simulink model "sfcndemo_vsfunc"  (Simulink 7.6)
settings: Solver=ode45  StartTime=0.0  StopTime=50  RelTol=1e-3
Description:
  | Continuous-Time Variable Step S-function
settings Model: Creator=The MathWorks Inc.  ExtModeTrigMode=oneshot  ExtModeArmWhenConnect=off  ExtModeAutoUpdateStatusClock=off
settings DataIOCC: LimitDataPoints=off  SaveFormat=StructureWithTime  SaveState=on  OutputSaveName=yout1
settings OptimizationCC: BlockReduction=off  BooleanDataType=off  InlineInvariantSignals=on  InitFltsAndDblsToZero=on
settings DebuggingCC: SaveWithParameterizedLinksMsg=none  SignalResolutionControl=TryResolveAllWithWarning  SolverPrmCheckMsg=none  MultiTaskDSMMsg=warning  MultiTaskCondExecSysMsg=none
settings HardwareCC: TargetUnknown=on
settings RTWCC: IncludeERTFirstTime=on
settings CodeAppCC: CustomSymbolStrFcn=$F$N$M
settings GRTTargetCC: TargetFcnLib=ansi_tfl_tmw.mat

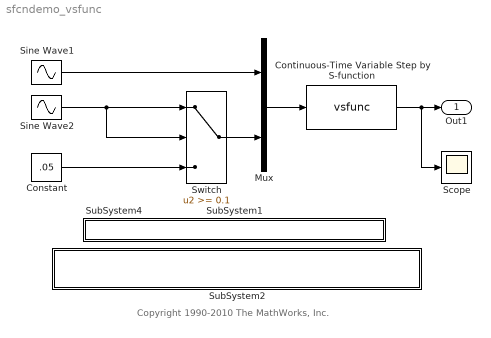
== system sfcndemo_vsfunc ==
  note: Copyright 1990-2010 The MathWorks, Inc.
  Constant : Constant  Value=.05
  Continuous-Time Variable Step by S-function : S-Function  FunctionName=vsfunc  EnableBusSupport=off
      mask Display: disp('dt           = u(2)\ny(t + dt) = u(t)')
  Mux : Mux  Inputs=2
  Scope : Scope
      settings: TimeRange=50  YMin=-1  YMax=1  SaveName=scopeout1
  Sine Wave1 : Sin  Frequency=2*pi  SampleTime=0
  Sine Wave2 : Sin  Amplitude=2  Frequency=2*pi  SampleTime=0
  SubSystem1 : Subsystem  mask{filename=vsfunc.c}
      mask init:
      | x=sfundemo_maskdisp;
      settings: AttributesFormatString=\n  OpenFcn=sfundemo_openfcn
      mask Display: disp(x);
  SubSystem2 : Subsystem  mask{filename=vsfunc.m}
      mask init:
      | x=sfundemo_maskdisp;
      settings: AttributesFormatString=\n  OpenFcn=sfundemo_openfcn
      mask Display: disp(['MATLAB file: ' x '\nNote:to run this file, please disable the executable mex file in your path.']);
  SubSystem4 : Subsystem  mask{filename=vsfunc.m}
      mask init:
      | x=sfundemo_maskdisp;
      settings: AttributesFormatString=\n  OpenFcn=sfundemo_openfcn
      mask Display: disp(x);
  Switch : Switch  Threshold=0.1  SaturateOnIntegerOverflow=on  InputSameDT=on
  Out1 : Outport  InitialOutput=0
  wires:
  Constant/1 -> Switch/3
  Mux/1 -> Continuous-Time Variable Step by S-function/1
  Sine Wave2/1 -> Switch/1, Switch/2
  Continuous-Time Variable Step by S-function/1 -> Out1/1, Scope/1
  Sine Wave1/1 -> Mux/1
  Switch/1 -> Mux/2

== system sfcndemo_vsfunc/SubSystem1 ==

== system sfcndemo_vsfunc/SubSystem2 ==

== system sfcndemo_vsfunc/SubSystem4 ==
